simulink model "auto"  (R2024b)
settings: Solver=VariableStepAuto  StartTime=0.0  StopTime=10.0  RelTol=1e-3
undefined symbols (not defined in the file): control, controlParams, ControlSampleTime, Cruise_a, flightState, FSState, FWControlParams, FWTrimSpeed, uavParam, Vt, w_trim, zGround
libraries: slpidlib x21, simulink x6, uavalgslib x6
(part 1 of 4)
settings Model: Creator=USER  LastModifiedBy=USER

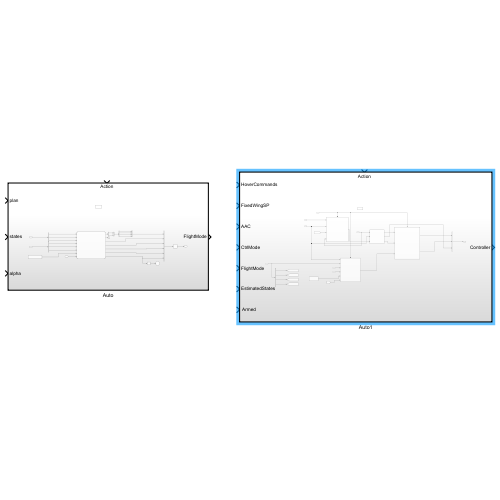
[thumbnail: Simulink's stored preview of the top-level diagram]
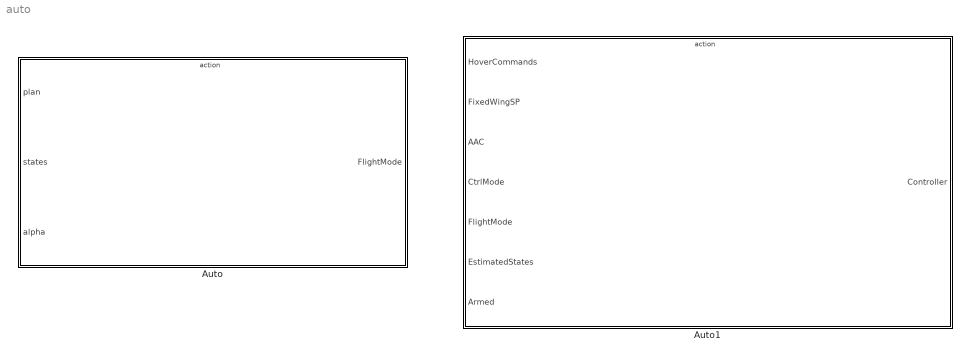
== system auto ==
  Auto : Subsystem  TreatAsAtomicUnit=on
  Auto1 : Subsystem  TreatAsAtomicUnit=on

== system auto/Auto ==
  plan : Inport  OutDataTypeStr=Bus: plan  SampleTime=0.005
  states : Inport  Port=2  OutDataTypeStr=Bus: states  SampleTime=0.005
  alpha : Inport  Port=3  SampleTime=0.005
  Action Port : ActionPort
  Bus Creator : BusCreator  Inputs=4  OutDataTypeStr=Bus: HoverSPBus
      settings: InheritFromInputs=off
  Bus Creator1 : BusCreator  Inputs=6  OutDataTypeStr=Bus: flightmode
  Bus Selector : BusSelector  OutputSignals=LAP,YawCmd
  Bus Selector1 : BusSelector  OutputSignals=mode,ToWP,FromWP
  Bus Selector2 : BusSelector  OutputSignals=pose,states,ground
  Compare To Constant : simulink/Logic and Bit Operations/Compare To Constant  relop===  const=2  OutDataTypeStr=boolean
  Constant2 : Constant  Value=FSState  SampleTime=-1
  Demux : Demux
  Guidance Mode Selector : Stateflow chart  TreatAsAtomicUnit=on
      settings: PortSchema="{\"entries\":[{\"content\":{\"sides\":[{\"content\":{\"connectorIds\":[\"In1\",\"In2\",\"In3\",\"In4\",\"In5\",\"In7\",\"In6\",\"In8\"]},\"type\":\"ConnectorPlacement.EquallySpacedRectSide\",\"uuid\":\"a9cfd0e2-196c-422d-b359-9161a47768c9\"},{\"content\":{\"connectorIds\":[\"Out7\",\"Out2\",\"Out4\",\"Out3\",\"Out5\",\"Out6\",\"Out1\"],\"side\":\"RIGHT\"},\"type\":\"ConnectorPlacement.EquallySpacedRectSide\",\"uuid\":\"4fed41ae-e7cf-4de3-8bdb-9e24e7d8b079\"},{\"content\":{\"side\":\"TOP\"},\"type\":\"ConnectorPlacement.EquallySpacedRectSide\",\"uuid\":\"2d49ff20-2f63-498d-ac9d-820eae01f794\"},{\"content\":{\"side\":\"BOTTOM\"},\"type\":\"ConnectorPlacement.EquallySpacedRectSide\",\"uuid\":\"da24ee44-6e15-4e50-9b36-ff21cb47946d\"}]},\"type\":\"ConnectorPlacement.EquallySpacedConnector\",\"uuid\":\"88d403f4-ad96-40f9-9697-84906f26a8bf\"}],\"packageUris\":[\"http://schema.mathworks.com/mf0/Connector/R2020b\"],\"version\":\"1.0\"}"
  Mux : Mux  Inputs=2
  Stop Simulation : Stop
  Terminator : Terminator
  Unit Delay : UnitDelay  SampleTime=-1  HasFrameUpgradeWarning=on
  FlightMode : Outport  OutDataTypeStr=Bus: flightmode
  wires:
  Bus Selector1/1 -> Guidance Mode Selector/1(mode)  "<mode>"
  Guidance Mode Selector/6(FlightMode) -> Bus Creator1/5  "FlightMode"
  Bus Selector1/3 -> Guidance Mode Selector/3(FromWP)  "<FromWP>"
  Bus Selector2/3 -> Guidance Mode Selector/7(Ground)  "<ground>"
  Bus Selector/1 -> Mux/1  "<LAP>"
  Guidance Mode Selector/5(controlMode) -> Bus Creator1/4  "controlMode"
  Guidance Mode Selector/3(aacSP) -> Bus Creator1/3  "AACSP"
  Guidance Mode Selector/7(InnerLoopCmds) -> Bus Selector/1
  Guidance Mode Selector/2(GdncMode) -> Terminator/1
  Bus Selector/2 -> Mux/2  "<YawCmd>"
  Compare To Constant/1 -> Stop Simulation/1
  Bus Selector2/2 -> Guidance Mode Selector/5(States)  "<states>"
  Mux/1 -> Demux/1
  Bus Selector2/1 -> Guidance Mode Selector/4(Pose)  "<pose>"
  Guidance Mode Selector/1(Status) -> Compare To Constant/1, Bus Creator1/6  "Status"
  Guidance Mode Selector/4(FixedWingSP) -> Bus Creator1/2  "FixedWingSP"
  Bus Selector1/2 -> Guidance Mode Selector/2(ToWP)  "<ToWP>"
  Demux/1 -> Bus Creator/1  "X"
  Demux/2 -> Bus Creator/2  "Y"
  Demux/3 -> Bus Creator/3  "Z"
  Demux/4 -> Bus Creator/4  "Yaw"
  Bus Creator/1 -> Bus Creator1/1  "HoverSP"
  Bus Creator1/1 -> Unit Delay/1
  alpha/1 -> Guidance Mode Selector/8(a)
  Constant2/1 -> Guidance Mode Selector/6(PresetMode)
  states/1 -> Bus Selector2/1
  plan/1 -> Bus Selector1/1
  Unit Delay/1 -> FlightMode/1

== system auto/Auto1 ==
  HoverCommands : Inport  OutDataTypeStr=Bus: HoverSPBus
  FixedWingSP : Inport  Port=2
  AAC : Inport  Port=3
  CtrlMode : Inport  Port=4
  FlightMode : Inport  Port=5
  EstimatedStates : Inport  Port=6
  " Armed" : Inport  Port=7
  Action Port : ActionPort
  Blend Scheduler : Subsystem
  Bus Creator : BusCreator  Inputs=3  OutDataTypeStr=Bus: controller
  Bus Selector2 : BusSelector  OutputSignals=inTransition,TransitionCondition,BackTransitionCondition,TransitionStep
  Fixed Wing Controller : Subsystem  TreatAsAtomicUnit=on  VariantControl=Fixed Wing Controller
  Manual Control : Subsystem
  Multicopter Controller : Subsystem  TreatAsAtomicUnit=on
  Scheduler : Subsystem  SystemSampleTime=0.005
  Controller : Outport
  wires:
  Scheduler/1(MotorActuatorCommands) -> Bus Creator/1  "MotorActuatorCommands"
  Manual Control/1(AERT) -> Fixed Wing Controller/5(AERT)
  Scheduler/2(CtrlSurfaceCommands) -> Bus Creator/2  "CtrlSurfaceCommands"
  Fixed Wing Controller/1(Actuator) -> Scheduler/3(FixedWingActuators)
  Blend Scheduler/2(alpha) -> Bus Creator/3  "a"
  Multicopter Controller/1(MixerCommands) -> Blend Scheduler/3(MixerCommands)
  AAC/1 -> Fixed Wing Controller/3(AAC SP)
  FixedWingSP/1 -> Fixed Wing Controller/4(FixedWingSP)
  [InTransition] -> Multicopter Controller/3(InTransition)
  " Armed"/1 -> Fixed Wing Controller/Enable, Scheduler/Enable, Multicopter Controller/Enable
  HoverCommands/1 -> Multicopter Controller/1(Hover Commands)
  EstimatedStates/1 -> Fixed Wing Controller/1(States), Blend Scheduler/2(States), Multicopter Controller/2(States)
  FlightMode/1 -> Multicopter Controller/4(FlightMode), Blend Scheduler/1(FlightMode)
  Bus Selector2/2 -> [TransitionDone]  "<TransitionCondition>"
  CtrlMode/1 -> Bus Selector2/1, Fixed Wing Controller/2(Control Mode)
  Bus Selector2/1 -> [InTransition]  "<inTransition>"
  Bus Selector2/3 -> [BackTransitionDone]  "<BackTransitionCondition>"
  Bus Creator/1 -> Controller/1
  Blend Scheduler/3(FlightState) -> Scheduler/2(FlightState)
  [InTransition] -> Fixed Wing Controller/6(In1)
  Bus Selector2/4 -> [TransitionStep]  "<TransitionStep>"
  Blend Scheduler/1(MotorCommands) -> Scheduler/1(MotorCommands)

== system auto/Auto/Guidance Mode Selector/GuidanceLogic.BackTransition ==
  States : Inport  OutDataTypeStr=Bus: GuidanceStates
  Action Port : ActionPort
      settings: CopyFcn=Stateflow.SLINSF.SimulinkMan.removeBlockPreDeleteFcn  PreDeleteFcn=Stateflow.SLINSF.SimulinkMan.unsafePredeleteFcn
  Bus Creator1 : BusCreator  Inputs=3  OutDataTypeStr=Bus: innerLoopCmdsBus  NonVirtualBus=on
  Bus Selector : BusSelector  OutputSignals=Xe
  Constant : Constant  Value=0
  Constant1 : Constant  Value=0
  Constant2 : Constant  Value=0
  Data Type Conversion : DataTypeConversion  OutDataTypeStr=uint8  SaturateOnIntegerOverflow=off  RndMeth=Floor
  Gain : Gain
  Status : Outport
  InnerLoopCmds : Outport  Port=2  OutDataTypeStr=Bus: innerLoopCmdsBus
  wires:
  States/1 -> Bus Selector/1
  Bus Selector/1 -> Gain/1  "<Xe>"
  Bus Creator1/1 -> InnerLoopCmds/1
  Constant1/1 -> Bus Creator1/2  "HeadingCmd"
  Constant2/1 -> Bus Creator1/3  "YawCmd"
  Data Type Conversion/1 -> Status/1
  Gain/1 -> Bus Creator1/1  "LAP"
  Constant/1 -> Data Type Conversion/1

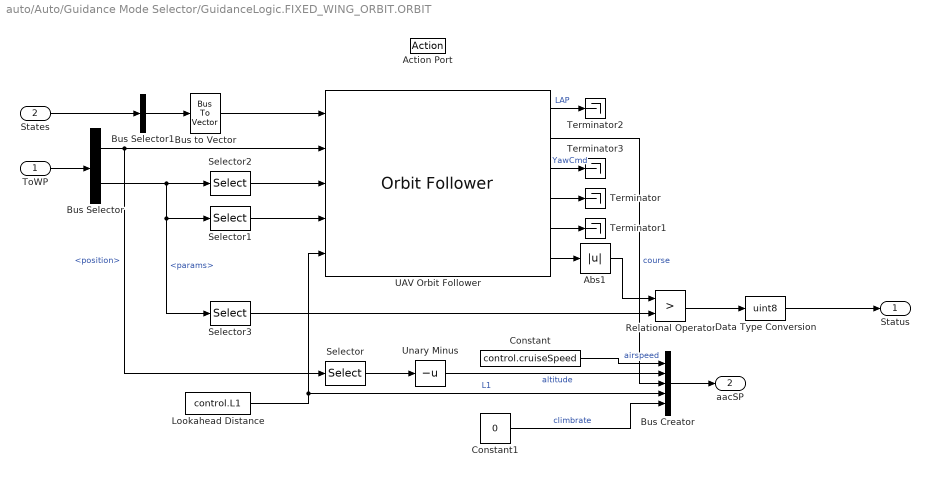
== system auto/Auto/Guidance Mode Selector/GuidanceLogic.FIXED_WING_ORBIT.ORBIT ==
  ToWP : Inport  OutDataTypeStr=Bus: UAVPathManagerBus
  States : Inport  Port=2
  Action Port : ActionPort
      settings: CopyFcn=Stateflow.SLINSF.SimulinkMan.removeBlockPreDeleteFcn  PreDeleteFcn=Stateflow.SLINSF.SimulinkMan.unsafePredeleteFcn
  Abs1 : Abs  SaturateOnIntegerOverflow=off
  Bus Creator : BusCreator  Inputs=5  OutDataTypeStr=Bus: AAC  NonVirtualBus=on
      settings: InheritFromInputs=off
  Bus Selector : BusSelector  OutputSignals=position,params
  Bus Selector1 : BusSelector  OutputSignals=Xe,course  OutputAsBus=on
  Bus to Vector : BusToVector
  Constant : Constant  Value=control.cruiseSpeed
  Constant1 : Constant  Value=0
  Data Type Conversion : DataTypeConversion  OutDataTypeStr=uint8  SaturateOnIntegerOverflow=off  RndMeth=Floor
  Lookahead Distance : Constant  Value=control.L1  OutDataTypeStr=double
  Relational Operator : RelationalOperator  Operator=>  OutDataTypeStr=boolean  RndMeth=Simplest  InputSameDT=off
  Selector : Selector  InputPortWidth=3  IndexOptions=Index vector (dialog)  Indices=3  OutputSizes=1
  Selector1 : Selector  InputPortWidth=4  IndexOptions=Index vector (dialog)  Indices=2  OutputSizes=1
  Selector2 : Selector  InputPortWidth=4  IndexOptions=Index vector (dialog)  Indices=1  OutputSizes=1
  Selector3 : Selector  InputPortWidth=4  IndexOptions=Index vector (dialog)  Indices=3  OutputSizes=1
  Terminator{,1..3} (4 alike) : Terminator
  UAV Orbit Follower : uavalgslib/Orbit Follower  UAVType=fixed-wing  MinOrbitRadius=control.turningRadius  MinLookaheadDistance=control.L1  ExternalReset=none  ShowCrossTrackErrorOutput=off  ShowNumTurnsOutput=on  SimulateUsing=Code generation
  Unary Minus : UnaryMinus
  Status : Outport
  aacSP : Outport  Port=2
  wires:
  Bus to Vector/1 -> UAV Orbit Follower/1
  Selector2/1 -> UAV Orbit Follower/3
  Bus Selector/1 -> UAV Orbit Follower/2, Selector/1  "<position>"
  ToWP/1 -> Bus Selector/1
  Bus Selector/2 -> Selector1/1, Selector3/1, Selector2/1  "<params>"
  Selector3/1 -> Relational Operator/2
  Relational Operator/1 -> Data Type Conversion/1
  UAV Orbit Follower/4 -> Terminator/1
  UAV Orbit Follower/5 -> Terminator1/1
  Bus Selector1/1 -> Bus to Vector/1
  States/1 -> Bus Selector1/1
  UAV Orbit Follower/1 -> Terminator2/1  "LAP"
  Lookahead Distance/1 -> UAV Orbit Follower/5, Bus Creator/4  "L1"
  Bus Creator/1 -> aacSP/1
  UAV Orbit Follower/2 -> Bus Creator/3  "course"
  Constant/1 -> Bus Creator/1  "airspeed"
  Unary Minus/1 -> Bus Creator/2  "altitude"
  UAV Orbit Follower/3 -> Terminator3/1  "YawCmd"
  Selector/1 -> Unary Minus/1
  UAV Orbit Follower/6 -> Abs1/1
  Abs1/1 -> Relational Operator/1
  Selector1/1 -> UAV Orbit Follower/4
  Constant1/1 -> Bus Creator/5  "climbrate"
  Data Type Conversion/1 -> Status/1

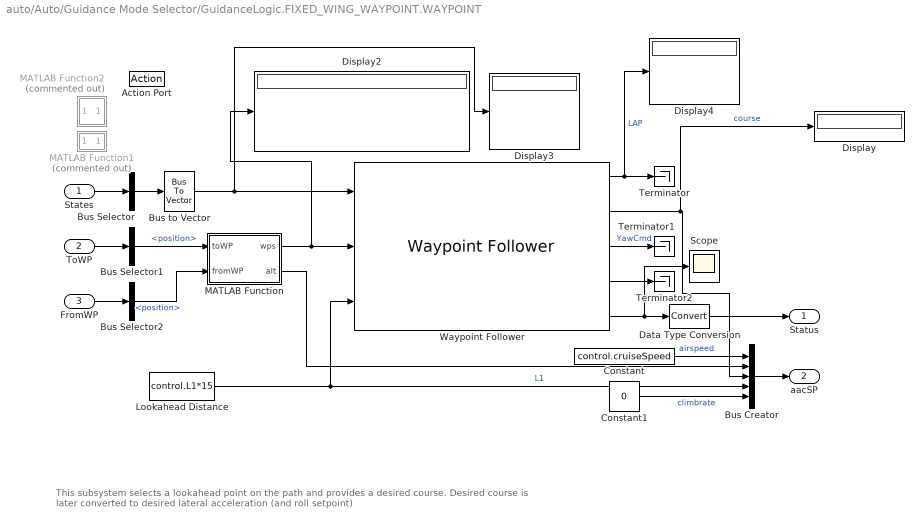
== system auto/Auto/Guidance Mode Selector/GuidanceLogic.FIXED_WING_WAYPOINT.WAYPOINT ==
  note: This subsystem selects a lookahead point on the path and provides a desired course. Desired course is later converted to desired lateral acceleration (and roll setpoint)
  States : Inport  OutDataTypeStr=Bus: GuidanceStates
  ToWP : Inport  Port=2  OutDataTypeStr=Bus: UAVPathManagerBus
  FromWP : Inport  Port=3  OutDataTypeStr=Bus: UAVPathManagerBus
  Action Port : ActionPort
      settings: CopyFcn=Stateflow.SLINSF.SimulinkMan.removeBlockPreDeleteFcn  PreDeleteFcn=Stateflow.SLINSF.SimulinkMan.unsafePredeleteFcn
  Bus Creator : BusCreator  Inputs=5  OutDataTypeStr=Bus: AAC  NonVirtualBus=on
      settings: InheritFromInputs=off
  Bus Selector : BusSelector  OutputSignals=Xe,course  OutputAsBus=on
  Bus Selector1 : BusSelector  OutputSignals=position
  Bus Selector2 : BusSelector  OutputSignals=position
  Bus to Vector : BusToVector
  Constant : Constant  Value=control.cruiseSpeed
  Constant1 : Constant  Value=0
  Data Type Conversion : DataTypeConversion  SaturateOnIntegerOverflow=off  RndMeth=Floor
  Display{,2..4} (4 alike) : Display
  Lookahead Distance : Constant  Value=control.L1*15  OutDataTypeStr=double
  MATLAB Function : MATLAB Function  TreatAsAtomicUnit=on
  MATLAB Function1 : MATLAB Function  Commented=on  TreatAsAtomicUnit=on
  MATLAB Function2 : MATLAB Function  Commented=on  TreatAsAtomicUnit=on
  Scope : Scope
  Terminator : Terminator
  Terminator1 : Terminator
  Terminator2 : Terminator
  Waypoint Follower : uavalgslib/Waypoint Follower  UAVType=fixed-wing  StartFrom=first  TransitionRadiusSource=internal  TransitionRadius=FWControl.transitionRadius  MinLookaheadDistance=control.L1  HoverAtLastWaypoint=off  YawInput=off  ShowCrossTrackErrorOutput=off  ShowStatusOutput=on  SimulateUsing=Code generation
  Status : Outport
  aacSP : Outport  Port=2
  wires:
  Lookahead Distance/1 -> Waypoint Follower/3, Bus Creator/4  "L1"
  Waypoint Follower/1 -> Display4/1, Terminator/1  "LAP"
  Waypoint Follower/3 -> Terminator1/1  "YawCmd"
  Waypoint Follower/4 -> Terminator2/1
  Constant/1 -> Bus Creator/1  "airspeed"
  States/1 -> Bus Selector/1
  Bus Selector/1 -> Bus to Vector/1
  Waypoint Follower/5 -> Scope/1, Data Type Conversion/1
  Data Type Conversion/1 -> Status/1
  Bus Creator/1 -> aacSP/1
  ToWP/1 -> Bus Selector1/1
  FromWP/1 -> Bus Selector2/1
  Bus Selector1/1 -> MATLAB Function/1(toWP)  "<position>"
  Bus Selector2/1 -> MATLAB Function/2(fromWP)  "<position>"
  MATLAB Function/2(alt) -> Bus Creator/2
  Waypoint Follower/2 -> Display/1, Bus Creator/3  "course"
  Constant1/1 -> Bus Creator/5  "climbrate"
  Bus to Vector/1 -> Display3/1, Waypoint Follower/1
  MATLAB Function/1(wps) -> Display2/1, Waypoint Follower/2

== system auto/Auto/Guidance Mode Selector/GuidanceLogic.ForwardTransition ==
  ToWP : Inport  OutDataTypeStr=Bus: UAVPathManagerBus
  FromWP : Inport  Port=2  OutDataTypeStr=Bus: UAVPathManagerBus
  Action Port : ActionPort
      settings: CopyFcn=Stateflow.SLINSF.SimulinkMan.removeBlockPreDeleteFcn  PreDeleteFcn=Stateflow.SLINSF.SimulinkMan.unsafePredeleteFcn
  Bus Creator : BusCreator  Inputs=5  OutDataTypeStr=Bus: AAC  NonVirtualBus=on
      settings: InheritFromInputs=off
  Bus Creator1 : BusCreator  Inputs=3  OutDataTypeStr=Bus: innerLoopCmdsBus  NonVirtualBus=on
  Bus Selector1 : BusSelector  OutputSignals=position
  Bus Selector2 : BusSelector  OutputSignals=position
  Constant : Constant  Value=0
  Constant1 : Constant  Value=0
  Constant2 : Constant  Value=0
  Constant3 : Constant  Value=[0 0 0]
  Data Type Conversion : DataTypeConversion  OutDataTypeStr=uint8  SaturateOnIntegerOverflow=off  RndMeth=Floor
  MATLAB Function : MATLAB Function  TreatAsAtomicUnit=on
  Switch : Switch  Criteria=u2 > Threshold  SaturateOnIntegerOverflow=off  InputSameDT=off
  Terminator : Terminator
  Status : Outport
  InnerLoopCmds : Outport  Port=2  OutDataTypeStr=Bus: innerLoopCmdsBus
  aacSP : Outport  Port=3
  wires:
  Bus Creator1/1 -> InnerLoopCmds/1
  Constant1/1 -> Bus Creator1/2  "HeadingCmd"
  Constant2/1 -> Bus Creator1/3  "YawCmd"
  Data Type Conversion/1 -> Status/1
  Constant/1 -> Data Type Conversion/1
  Constant3/1 -> Bus Creator1/1  "LAP"
  FromWP/1 -> Bus Selector2/1
  Bus Selector1/1 -> MATLAB Function/1(toWP)  "<position>"
  Bus Selector2/1 -> MATLAB Function/2(fromWP)  "<position>"
  ToWP/1 -> Bus Selector1/1
  Bus Creator/1 -> aacSP/1
  MATLAB Function/1(wps) -> Terminator/1
  MATLAB Function/2(alt) -> Bus Creator/2  "alt"

== system auto/Auto/Guidance Mode Selector/GuidanceLogic.Land.Descend ==
  ToWP : Inport  OutDataTypeStr=Bus: UAVPathManagerBus
  Ground : Inport  Port=2
  Pose : Inport  Port=3
  FromWP : Inport  Port=4  OutDataTypeStr=Bus: UAVPathManagerBus
  Action Port : ActionPort
      settings: CopyFcn=Stateflow.SLINSF.SimulinkMan.removeBlockPreDeleteFcn  PreDeleteFcn=Stateflow.SLINSF.SimulinkMan.unsafePredeleteFcn
  Bus Creator : BusCreator  Inputs=3  OutDataTypeStr=Bus: innerLoopCmdsBus  NonVirtualBus=on
      settings: InheritFromInputs=off
  Bus Selector : BusSelector  OutputSignals=position,params
  Constant : Constant  Value=3
  Constant3 : Constant  Value=0  OutDataTypeStr=uint8
  Hdg Cmd Sat : Saturate  UpperLimit=pi  LowerLimit=-pi
      settings: AttributesFormatString=[%<UpperLimit> %<LowerLimit>]
  MATLAB Function : MATLAB Function  TreatAsAtomicUnit=on
  Mux : Mux  Inputs=2
  Selector : Selector  InputPortWidth=3  IndexOptions=Index vector (dialog)  Indices=[1 2]  OutputSizes=1
  Selector1 : Selector  InputPortWidth=4  IndexOptions=Index vector (dialog)  Indices=4  OutputSizes=1
  Selector3 : Selector  InputPortWidth=4  IndexOptions=Index vector (dialog)  Indices=4  OutputSizes=1
  Waypoint Follower : uavalgslib/Waypoint Follower  UAVType=multirotor  StartFrom=first  TransitionRadiusSource=internal  TransitionRadius=1  MinLookaheadDistance=0.1  HoverAtLastWaypoint=on  YawInput=on  ShowCrossTrackErrorOutput=off  ShowStatusOutput=off  SimulateUsing=Code generation
  Yaw Cmd Sat : Saturate  UpperLimit=pi  LowerLimit=-pi
      settings: AttributesFormatString=[%<UpperLimit> %<LowerLimit>]
  InnerLoopCmds : Outport  OutDataTypeStr=Bus: innerLoopCmdsBus
  Status : Outport  Port=2
  wires:
  Bus Creator/1 -> InnerLoopCmds/1
  Bus Selector/1 -> Selector/1  "<position>"
  Yaw Cmd Sat/1 -> Bus Creator/3  "YawCmd"
  Hdg Cmd Sat/1 -> Bus Creator/2  "HeadingCmd"
  ToWP/1 -> Bus Selector/1
  Selector1/1 -> Yaw Cmd Sat/1
  Selector3/1 -> Hdg Cmd Sat/1
  Selector/1 -> Mux/1  "LAP"
  Bus Selector/2 -> MATLAB Function/3(ToWPParam), Selector1/1, Selector3/1  "<params>"
  Ground/1 -> Mux/2
  Constant3/1 -> Status/1
  Mux/1 -> MATLAB Function/2(ToWPPos)  "LAP"
  FromWP/1 -> MATLAB Function/1(FromWP)
  Pose/1 -> Waypoint Follower/1
  MATLAB Function/1(wps) -> Waypoint Follower/2
  Constant/1 -> Waypoint Follower/3
  Waypoint Follower/1 -> Bus Creator/1  "LAP"

== system auto/Auto/Guidance Mode Selector/GuidanceLogic.Land.ToLand ==
  Pose : Inport
  ToWP : Inport  Port=2  OutDataTypeStr=Bus: UAVPathManagerBus
  FromWP : Inport  Port=3  OutDataTypeStr=Bus: UAVPathManagerBus
  Action Port : ActionPort
      settings: CopyFcn=Stateflow.SLINSF.SimulinkMan.removeBlockPreDeleteFcn  PreDeleteFcn=Stateflow.SLINSF.SimulinkMan.unsafePredeleteFcn
  Bus Creator1 : BusCreator  Inputs=3  OutDataTypeStr=Bus: innerLoopCmdsBus  NonVirtualBus=on
  Constant : Constant  Value=0  OutDataTypeStr=uint8
  Lookahead Distance : Constant  Value=10  OutDataTypeStr=double
  MATLAB Function : MATLAB Function  TreatAsAtomicUnit=on
  Scope : Scope
  Waypoint Follower : uavalgslib/Waypoint Follower  UAVType=multirotor  StartFrom=first  TransitionRadiusSource=internal  TransitionRadius=1  MinLookaheadDistance=0.1  HoverAtLastWaypoint=on  YawInput=on  ShowCrossTrackErrorOutput=off  ShowStatusOutput=off  SimulateUsing=Code generation
  Status : Outport
  InnerLoopCmds : Outport  Port=2  OutDataTypeStr=Bus: innerLoopCmdsBus
  wires:
  Constant/1 -> Status/1
  MATLAB Function/1(wps) -> Waypoint Follower/2
  Lookahead Distance/1 -> Waypoint Follower/3
  Bus Creator1/1 -> InnerLoopCmds/1
  ToWP/1 -> MATLAB Function/2(ToWP)
  Waypoint Follower/2 -> Bus Creator1/2  "HeadingCmd"
  FromWP/1 -> MATLAB Function/1(FromWP)
  Waypoint Follower/4 -> Scope/1
  Pose/1 -> Waypoint Follower/1
  Waypoint Follower/3 -> Bus Creator1/3  "YawCmd"
  Waypoint Follower/1 -> Bus Creator1/1  "LAP"

== system auto/Auto/Guidance Mode Selector/GuidanceLogic.Orbit ==
  ToWP : Inport  OutDataTypeStr=Bus: UAVPathManagerBus
  Pose : Inport  Port=2
  Action Port : ActionPort
      settings: CopyFcn=Stateflow.SLINSF.SimulinkMan.removeBlockPreDeleteFcn  PreDeleteFcn=Stateflow.SLINSF.SimulinkMan.unsafePredeleteFcn
  Abs : Abs  SaturateOnIntegerOverflow=off
  Bus Creator : BusCreator  Inputs=3  OutDataTypeStr=Bus: innerLoopCmdsBus  NonVirtualBus=on
  Bus Selector : BusSelector  OutputSignals=position,params
  Data Type Conversion : DataTypeConversion  OutDataTypeStr=uint8  SaturateOnIntegerOverflow=off  RndMeth=Floor
  Lookahead Distance : Constant  Value=5  OutDataTypeStr=double
  Radius : Selector  InputPortWidth=4  IndexOptions=Index vector (dialog)  Indices=[3]  OutputSizes=1
  Relational Operator : RelationalOperator  Operator=>  OutDataTypeStr=boolean  RndMeth=Simplest  InputSameDT=off
  Sign : Signum  ZeroCross=off
  Terminator : Terminator
  Terminator1 : Terminator
  Turns : Selector  InputPortWidth=4  IndexOptions=Index vector (dialog)  Indices=[1]  OutputSizes=1
  UAV Orbit Follower : uavalgslib/Orbit Follower  UAVType=multirotor  MinOrbitRadius=1  MinLookaheadDistance=0.1  ExternalReset=none  ShowCrossTrackErrorOutput=off  ShowNumTurnsOutput=on  SimulateUsing=Code generation
  InnerLoopCmds : Outport  OutDataTypeStr=Bus: innerLoopCmdsBus
  Status : Outport  Port=2
  wires:
  Pose/1 -> UAV Orbit Follower/1
  Lookahead Distance/1 -> UAV Orbit Follower/5
  Abs/1 -> UAV Orbit Follower/3
  Bus Selector/1 -> UAV Orbit Follower/2  "<position>"
  ToWP/1 -> Bus Selector/1
  Bus Creator/1 -> InnerLoopCmds/1
  UAV Orbit Follower/2 -> Bus Creator/2  "HeadingCmd"
  UAV Orbit Follower/3 -> Bus Creator/3  "YawCmd"
  Bus Selector/2 -> Turns/1, Radius/1  "<params>"
  Radius/1 -> Abs/1, Sign/1
  Sign/1 -> UAV Orbit Follower/4
  Relational Operator/1 -> Data Type Conversion/1
  Turns/1 -> Relational Operator/2
  Data Type Conversion/1 -> Status/1
  UAV Orbit Follower/6 -> Relational Operator/1
  UAV Orbit Follower/4 -> Terminator/1
  UAV Orbit Follower/5 -> Terminator1/1
  UAV Orbit Follower/1 -> Bus Creator/1  "LAP"

== system auto/Auto/Guidance Mode Selector/GuidanceLogic.Takeoff ==
  ToWP : Inport  OutDataTypeStr=Bus: UAVPathManagerBus
  Pose : Inport  Port=2
  Action Port : ActionPort
      settings: CopyFcn=Stateflow.SLINSF.SimulinkMan.removeBlockPreDeleteFcn  PreDeleteFcn=Stateflow.SLINSF.SimulinkMan.unsafePredeleteFcn
  Bus Creator : BusCreator  Inputs=3  OutDataTypeStr=Bus: innerLoopCmdsBus  NonVirtualBus=on
      settings: InheritFromInputs=off
  Bus Selector : BusSelector  OutputSignals=position,params
  Constant : Constant  Value=0  OutDataTypeStr=uint8
  Constant1 : Constant  Value=0
  Demux : Demux  Outputs=[2 2]
  Demux1 : Demux  Outputs=[2 1]
  Hdg. Cmd Sat : Saturate  UpperLimit=pi  LowerLimit=-pi
      settings: AttributesFormatString=[%<UpperLimit> %<LowerLimit>]
  Mux : Mux  Inputs=2
  Selector3 : Selector  InputPortWidth=4  IndexOptions=Index vector (dialog)  Indices=4  OutputSizes=1
  Terminator : Terminator
  Terminator1 : Terminator
  Yaw Cmd Sat : Saturate  UpperLimit=pi  LowerLimit=-pi
      settings: AttributesFormatString=[%<UpperLimit> %<LowerLimit>]
  InnerLoopCmds : Outport  OutDataTypeStr=Bus: innerLoopCmdsBus
  Status : Outport  Port=2
  wires:
  Hdg. Cmd Sat/1 -> Bus Creator/2  "HeadingCmd"
  Bus Creator/1 -> InnerLoopCmds/1
  Constant/1 -> Status/1
  Pose/1 -> Demux/1
  Yaw Cmd Sat/1 -> Bus Creator/3  "YawCmd"
  ToWP/1 -> Bus Selector/1
  Bus Selector/2 -> Selector3/1  "<params>"
  Demux/1 -> Mux/1
  Bus Selector/1 -> Demux1/1  "<position>"
  Demux/2 -> Terminator/1
  Demux1/1 -> Terminator1/1
  Selector3/1 -> Hdg. Cmd Sat/1
  Constant1/1 -> Yaw Cmd Sat/1
  Demux1/2 -> Mux/2
  Mux/1 -> Bus Creator/1  "LAP"

== system auto/Auto/Guidance Mode Selector/GuidanceLogic.WP ==
  FromWP : Inport  OutDataTypeStr=Bus: UAVPathManagerBus
  Pose : Inport  Port=2
  ToWP : Inport  Port=3  OutDataTypeStr=Bus: UAVPathManagerBus
  Action Port : ActionPort
      settings: CopyFcn=Stateflow.SLINSF.SimulinkMan.removeBlockPreDeleteFcn  PreDeleteFcn=Stateflow.SLINSF.SimulinkMan.unsafePredeleteFcn
  Back Transition Guard : Subsystem
  Bus Creator : BusCreator  Inputs=3  OutDataTypeStr=Bus: innerLoopCmdsBus  NonVirtualBus=on
  Bus Creator1 : BusCreator  Inputs=1
  Bus Creator2 : BusCreator  Inputs=3
  Bus Selector : BusSelector  OutputSignals=position
  Constant1 : Constant
  Data Type Conversion : DataTypeConversion  OutDataTypeStr=uint8  SaturateOnIntegerOverflow=off  RndMeth=Floor
  Data Type Conversion1 : DataTypeConversion  OutDataTypeStr=double  SaturateOnIntegerOverflow=off  RndMeth=Floor
  Data Type Conversion2 : DataTypeConversion  OutDataTypeStr=double  SaturateOnIntegerOverflow=off  RndMeth=Floor
  Demux : Demux  Outputs=3
  Dist2WP : Subsystem
  Lookahead Distance : Constant  Value=10  OutDataTypeStr=double
  MATLAB Function : MATLAB Function  TreatAsAtomicUnit=on
  Relational Operator : RelationalOperator  OutDataTypeStr=boolean  RndMeth=Simplest  InputSameDT=off
  Scope : Scope
  Selector : Selector  InputPortWidth=3  IndexOptions=Index vector (dialog)  Indices=3  OutputSizes=1
  Terminator1 : Terminator
  Waypoint Follower : uavalgslib/Waypoint Follower  UAVType=multirotor  StartFrom=closest  TransitionRadiusSource=internal  TransitionRadius=R_WAYPOINTTRANSITION  MinLookaheadDistance=0.1  HoverAtLastWaypoint=off  YawInput=on  ShowCrossTrackErrorOutput=off  ShowStatusOutput=off  SimulateUsing=Code generation
  Yaw Cmd Sat : Saturate  UpperLimit=pi  LowerLimit=-pi
      settings: AttributesFormatString=[%<UpperLimit> %<LowerLimit>]
  InnerLoopCmds : Outport  OutDataTypeStr=Bus: innerLoopCmdsBus
  Status : Outport  Port=2
  wires:
  Data Type Conversion/1 -> Status/1
  Bus Creator/1 -> InnerLoopCmds/1
  ToWP/1 -> Dist2WP/3(ToWP), Bus Selector/1, MATLAB Function/2(ToWP)
  MATLAB Function/1(wps) -> Waypoint Follower/2
  Waypoint Follower/2 -> Bus Creator/2  "HeadingCmd"
  Waypoint Follower/4 -> Scope/1
  Dist2WP/1(Dist) -> Relational Operator/2
  FromWP/1 -> Back Transition Guard/2(FromWP)
  Relational Operator/1 -> Data Type Conversion/1
  Back Transition Guard/1(PrevWP) -> Dist2WP/2(FromWP), MATLAB Function/1(FromWP)
  Pose/1 -> Back Transition Guard/1(Poses), Waypoint Follower/1, Dist2WP/1(Pose)
  Lookahead Distance/1 -> Waypoint Follower/3
  Waypoint Follower/3 -> Yaw Cmd Sat/1  "YawCmd"
  Yaw Cmd Sat/1 -> Bus Creator/3  "YawCmd"
  Constant1/1 -> Relational Operator/1
  Bus Creator1/1 -> Data Type Conversion1/1  "LAP"
  Waypoint Follower/1 -> Demux/1  "LAP"
  Demux/3 -> Terminator1/1
  Data Type Conversion1/1 -> Selector/1  "LAP"
  Selector/1 -> Bus Creator2/3  "Z"
  Demux/1 -> Bus Creator2/1  "X"
  Demux/2 -> Bus Creator2/2  "Y"
  Bus Creator2/1 -> Data Type Conversion2/1  "LAP"
  Data Type Conversion2/1 -> Bus Creator/1  "LAP"
  Bus Selector/1 -> Bus Creator1/1  "<position>"

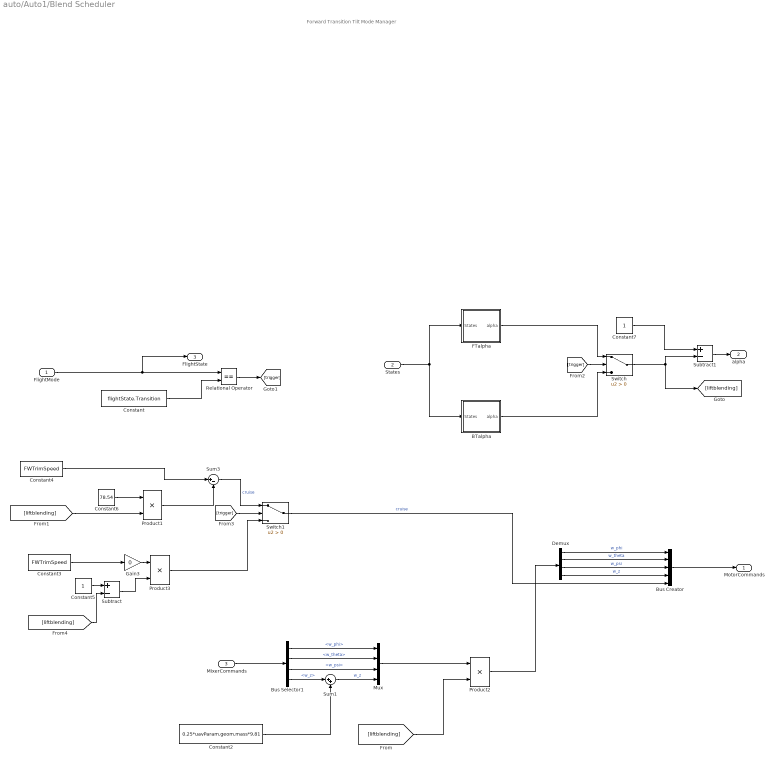
== system auto/Auto1/Blend Scheduler ==
  note: Forward Transition Tilt Mode Manager
  FlightMode : Inport
  States : Inport  Port=2
  MixerCommands : Inport  Port=3
  BTalpha : Subsystem  TreatAsAtomicUnit=on
  Bus Creator : BusCreator  Inputs=5
  Bus Selector1 : BusSelector  OutputSignals=w_phi,w_theta,w_psi,w_z
  Constant : Constant  Value=flightState.Transition
  Constant2 : Constant  Value=0.25*uavParam.geom.mass*9.81
  Constant3 : Constant  Value=FWTrimSpeed
  Constant4 : Constant  Value=FWTrimSpeed
  Constant5 : Constant
  Constant6 : Constant  Value=78.54
  Constant7 : Constant
  Demux : Demux
  FTalpha : Subsystem
  Gain3 : Gain  Gain=0
  Mux : Mux
  Product1 : Product
  Product2 : Product
  Product3 : Product
  Relational Operator : RelationalOperator  Operator===  OutDataTypeStr=boolean  RndMeth=Simplest  InputSameDT=off
  Subtract : Sum  Inputs=+-
  Subtract1 : Sum  Inputs=+-
  Sum1 : Sum  Inputs=|++
  Sum3 : Sum  Inputs=|+-
  Switch : Switch  Criteria=u2 > Threshold  SaturateOnIntegerOverflow=off  InputSameDT=off
  Switch1 : Switch  Criteria=u2 > Threshold  SaturateOnIntegerOverflow=off  InputSameDT=off
  MotorCommands : Outport
  alpha : Outport  Port=2
  FlightState : Outport  Port=3
  wires:
  FlightMode/1 -> Relational Operator/1, FlightState/1
  Relational Operator/1 -> [trigger]
  Bus Selector1/4 -> Sum1/1  "<w_z>"
  Constant2/1 -> Sum1/2
  [liftblending] -> Product2/2
  Mux/1 -> Product2/1
  MixerCommands/1 -> Bus Selector1/1
  Bus Selector1/1 -> Mux/1  "<w_phi>"
  Bus Selector1/2 -> Mux/2  "<w_theta>"
  Bus Selector1/3 -> Mux/3  "<w_psi>"
  Sum1/1 -> Mux/4  "w_z"
  Product2/1 -> Demux/1
  Demux/1 -> Bus Creator/1  "w_phi"
  Demux/2 -> Bus Creator/2  "w_theta"
  Demux/3 -> Bus Creator/3  "w_psi"
  Demux/4 -> Bus Creator/4  "w_z"
  Bus Creator/1 -> MotorCommands/1
  Constant6/1 -> Product1/1
  States/1 -> FTalpha/1(States), BTalpha/1(States)
  Switch/1 -> [liftblending], Subtract1/2
  FTalpha/1(alpha) -> Switch/1
  BTalpha/1(alpha) -> Switch/3
  [trigger] -> Switch/2
  Product1/1 -> Sum3/2
  Sum3/1 -> Switch1/1  "cruise"
  [trigger] -> Switch1/2
  Switch1/1 -> Bus Creator/5  "cruise"
  Constant3/1 -> Gain3/1
  Gain3/1 -> Product3/1
  Constant5/1 -> Subtract/1
  [liftblending] -> Subtract/2
  Subtract/1 -> Product3/2
  Product3/1 -> Switch1/3
  Constant7/1 -> Subtract1/1
  Subtract1/1 -> alpha/1
  Constant/1 -> Relational Operator/2
  [liftblending] -> Product1/2
  Constant4/1 -> Sum3/1

== system auto/Auto1/Fixed Wing Controller ==
  States : Inport
  Control Mode : Inport  Port=2
  AAC SP : Inport  Port=3  OutDataTypeStr=Bus: AAC
  FixedWingSP : Inport  Port=4  OutDataTypeStr=Bus: FixedWingCommandBus
  AERT : Inport  Port=5
  In1 : Inport  Port=6
  Actuator Armed : EnablePort
  Subsystem : Subsystem
  Actuator : Outport
  wires:
  States/1 -> Subsystem/1(States)
  Control Mode/1 -> Subsystem/2(Control Mode)
  AAC SP/1 -> Subsystem/3(AAC SP)
  Subsystem/1(Actuator) -> Actuator/1
  AERT/1 -> Subsystem/5(AERT)
  FixedWingSP/1 -> Subsystem/4(FixedWingSP)
  In1/1 -> Subsystem/6(Intransition)

== system auto/Auto1/Manual Control ==
  Bus Creator : BusCreator  Inputs=4
  Constant{,1..3} (4 alike) : Constant  Value=0  SampleTime=-1
  AERT : Outport
  wires:
  Constant/1 -> Bus Creator/1  "aileron"
  Constant1/1 -> Bus Creator/2  "throttle"
  Constant2/1 -> Bus Creator/3  "elevator"
  Constant3/1 -> Bus Creator/4  "rudder"
  Bus Creator/1 -> AERT/1

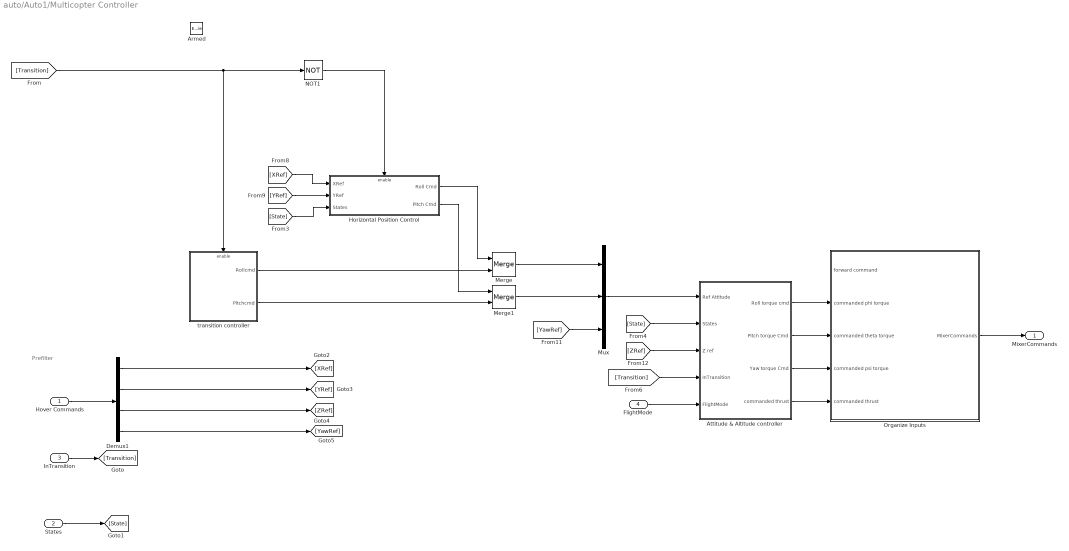
== system auto/Auto1/Multicopter Controller ==
  note: Prefilter
  Hover Commands : Inport  OutDataTypeStr=Bus: HoverSPBus
  States : Inport  Port=2
  InTransition : Inport  Port=3
  FlightMode : Inport  Port=4
  " Armed" : EnablePort
  Attitude & Altitude controller : Subsystem
  Demux1 : Demux
  Horizontal Position Control : Subsystem  TreatAsAtomicUnit=on
  Merge : Merge
  Merge1 : Merge
  Mux : Mux  Inputs=3
  NOT1 : Logic  Operator=NOT  IconShape=distinctive  AllPortsSameDT=off  OutDataTypeStr=boolean
  Organize Inputs : Subsystem
  transition controller : Subsystem
  MixerCommands : Outport
  wires:
  Organize Inputs/1(MixerCommands) -> MixerCommands/1
  Demux1/1 -> [XRef]
  [State] -> Horizontal Position Control/3(States)
  Demux1/3 -> [ZRef]
  NOT1/1 -> Horizontal Position Control/Enable
  [XRef] -> Horizontal Position Control/1(XRef)
  [YRef] -> Horizontal Position Control/2(YRef)
  InTransition/1 -> [Transition]
  States/1 -> [State]
  Hover Commands/1 -> Demux1/1
  Demux1/4 -> [YawRef]
  Mux/1 -> Attitude & Altitude controller/1(Ref Attitude)
  [State] -> Attitude & Altitude controller/2(States)
  [ZRef] -> Attitude & Altitude controller/3(Z ref)
  [Transition] -> Attitude & Altitude controller/4(InTransition)
  Attitude & Altitude controller/1(Roll torque cmd) -> Organize Inputs/2(commanded phi torque)
  Attitude & Altitude controller/2(Pitch torque Cmd) -> Organize Inputs/3(commanded theta torque)
  Attitude & Altitude controller/4(commanded thrust) -> Organize Inputs/5(commanded thrust)
  FlightMode/1 -> Attitude & Altitude controller/5(FlightMode)
  Attitude & Altitude controller/3(Yaw torque Cmd) -> Organize Inputs/4(commanded psi torque)
  [Transition] -> NOT1/1, transition controller/Enable
  [YawRef] -> Mux/3
  Demux1/2 -> [YRef]
  Merge/1 -> Mux/1
  Merge1/1 -> Mux/2
  transition controller/1(Rollcmd) -> Merge/2
  transition controller/2(Pitchcmd) -> Merge1/2
  Horizontal Position Control/1(Roll Cmd) -> Merge/1
  Horizontal Position Control/2(Pitch Cmd) -> Merge1/1

== system auto/Auto1/Scheduler ==
  MotorCommands : Inport
  FlightState : Inport  Port=2  OutDataTypeStr=Enum: flightState
  FixedWingActuators : Inport  Port=3
  " Armed" : EnablePort
  FixedWingScheduler : Subsystem
  Subsystem : Subsystem
  MotorActuatorCommands : Outport  OutputWhenDisabled=reset  InitialOutput=0
  CtrlSurfaceCommands : Outport  Port=2  OutDataTypeStr=Bus: FixedWingCtrlBus  OutputWhenDisabled=reset  InitialOutput=0  VectorParamsAs1DForOutWhenUnconnected=off
  wires:
  FixedWingScheduler/1(ActuatorControls) -> CtrlSurfaceCommands/1, Subsystem/2(FixedWingActuators)
  FlightState/1 -> Subsystem/1(FlightState), FixedWingScheduler/1(FlightState)
  Subsystem/1(ActuatorControls) -> MotorActuatorCommands/1
  MotorCommands/1 -> Subsystem/3(MotorCommands)
  FixedWingActuators/1 -> FixedWingScheduler/2(FixedWingActuators)

== system auto/Auto/Guidance Mode Selector/GuidanceLogic.WP/Back Transition Guard ==
  note: Set previous waypoint to current location if the UAV has just exited back transition
  Poses : Inport
  FromWP : Inport  Port=2
  Bus Selector : BusSelector  OutputSignals=mode
  Bus Selector1 : BusSelector  OutputSignals=position,params,mode
  Constant : Constant  Value=6
  Equal : RelationalOperator  Operator===  OutDataTypeStr=boolean  RndMeth=Simplest  InputSameDT=off
  Switch : Switch  Criteria=u2 > Threshold  SaturateOnIntegerOverflow=off  InputSameDT=off
  Triggered Subsystem : Subsystem  TreatAsAtomicUnit=on
  Out Bus Element2 : Outport  PortName=PrevWP  Element=mode
  Out Bus Element : Outport  PortName=PrevWP  Element=position
  Out Bus Element1 : Outport  PortName=PrevWP  Element=params
  wires:
  FromWP/1 -> Bus Selector1/1, Bus Selector/1
  Bus Selector/1 -> Equal/2  "<mode>"
  Constant/1 -> Equal/1
  Equal/1 -> Switch/2, Triggered Subsystem/Trigger
  Poses/1 -> Triggered Subsystem/1(Poses)
  Triggered Subsystem/1(HoldPositionValue) -> Switch/1
  Switch/1 -> Out Bus Element/1
  Bus Selector1/2 -> Out Bus Element1/1  "<params>"
  Bus Selector1/3 -> Out Bus Element2/1  "<mode>"
  Bus Selector1/1 -> Switch/3  "<position>"

== system auto/Auto/Guidance Mode Selector/GuidanceLogic.WP/Dist2WP ==
  Pose : Inport
  FromWP : Inport  Port=2
  ToWP : Inport  Port=3
  Bus Selector : BusSelector  OutputSignals=position
  Bus Selector1 : BusSelector  OutputSignals=position
  Demux : Demux  Outputs=[3 1]
  Dot Product : DotProduct  OutDataTypeStr=Inherit: Inherit via internal rule
  Subsystem : Subsystem
  Sum : Sum  Inputs=|-+
  Sum1 : Sum  Inputs=|+-
  Terminator : Terminator
  Dist : Outport
  wires:
  Sum1/1 -> Subsystem/1(V)
  Demux/2 -> Terminator/1
  Bus Selector/1 -> Sum/2, Sum1/1  "<position>"
  Demux/1 -> Sum/1
  Bus Selector1/1 -> Sum1/2  "<position>"
  Sum/1 -> Dot Product/1
  Subsystem/1(V_unit) -> Dot Product/2
  Pose/1 -> Demux/1
  Dot Product/1 -> Dist/1
  ToWP/1 -> Bus Selector/1
  FromWP/1 -> Bus Selector1/1

== system auto/Auto1/Blend Scheduler/BTalpha ==
  States : Inport
  Bus Selector : BusSelector  OutputSignals=airspeed
  Constant : Constant  Value=65
  Gain : Gain  Gain=1/20
  Saturation : Saturate  UpperLimit=1  LowerLimit=0
  Subtract : Sum  Inputs=+-
  alpha : Outport
  wires:
  Constant/1 -> Subtract/1
  Subtract/1 -> Gain/1
  Gain/1 -> Saturation/1
  Saturation/1 -> alpha/1
  States/1 -> Bus Selector/1
  Bus Selector/1 -> Subtract/2  "<airspeed>"

== system auto/Auto1/Blend Scheduler/FTalpha ==
  States : Inport
  1-a : Sum  Inputs=+-
  Bus Selector : BusSelector  OutputSignals=airspeed
  Constant3 : Constant  Value=35
  Constant5 : Constant  Value=Cruise_a
  Gain3 : Gain  Gain=1/10
  Saturation1 : Saturate  UpperLimit=10  LowerLimit=0
  Sum2 : Sum  Inputs=|+-
  alpha : Outport
  wires:
  1-a/1 -> alpha/1
  Bus Selector/1 -> Sum2/1  "<airspeed>"
  Gain3/1 -> 1-a/2
  Sum2/1 -> Saturation1/1
  Saturation1/1 -> Gain3/1
  Constant3/1 -> Sum2/2
  States/1 -> Bus Selector/1
  Constant5/1 -> 1-a/1

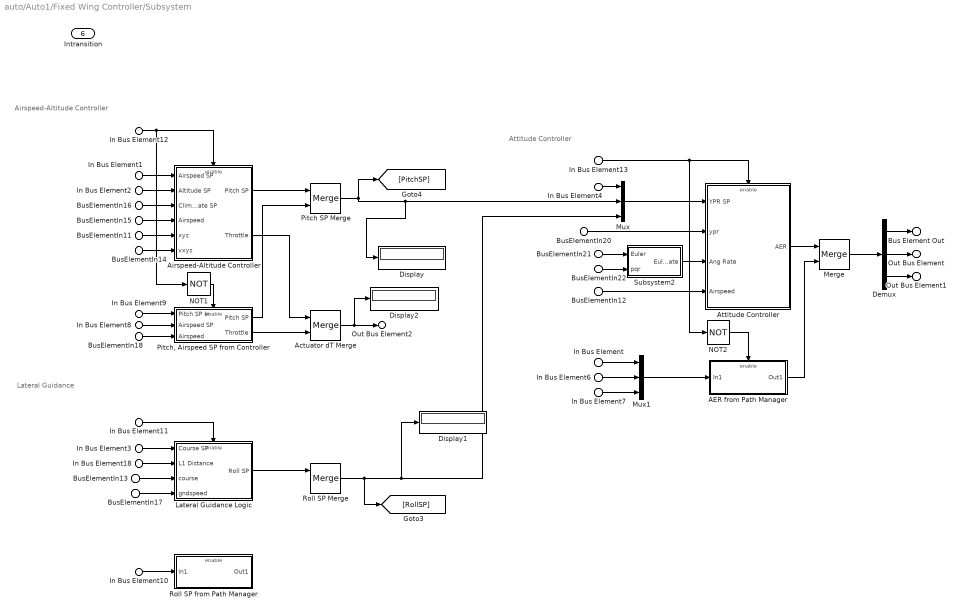
== system auto/Auto1/Fixed Wing Controller/Subsystem ==
  note: Airspeed-Altitude Controller
  note: Lateral Guidance
  note: Attitude Controller
  BusElementIn11 : Inport  PortName=States  Element=Xe
  BusElementIn12 : Inport  PortName=States  Element=airspeed
  BusElementIn15 : Inport  PortName=States  Element=airspeed
  BusElementIn18 : Inport  PortName=States  Element=airspeed
  BusElementIn13 : Inport  PortName=States  Element=course
  BusElementIn16 : Inport  PortName=States  Element=course
  BusElementIn14 : Inport  PortName=States  Element=Ve_ground
  BusElementIn17 : Inport  PortName=States  Element=gndspeed
  BusElementIn20 : Inport  PortName=States  Element=YPR
  BusElementIn21 : Inport  PortName=States  Element=Euler
  BusElementIn22 : Inport  PortName=States  Element=pqr
  In Bus Element11 : Inport  Port=2  PortName=Control Mode  Element=lateralGuidance
  In Bus Element12 : Inport  Port=2  PortName=Control Mode  Element=airspeedAltitude
  In Bus Element13 : Inport  Port=2  PortName=Control Mode  Element=attitude
  In Bus Element1 : Inport  Port=3  PortName=AAC SP  Element=airspeed
  In Bus Element2 : Inport  Port=3  PortName=AAC SP  Element=altitude
  In Bus Element18 : Inport  Port=3  PortName=AAC SP  Element=L1
  In Bus Element3 : Inport  Port=3  PortName=AAC SP  Element=course
  In Bus Element4 : Inport  Port=4  PortName=FixedWingSP  Element=yaw
  In Bus Element9 : Inport  Port=4  PortName=FixedWingSP  Element=pitch
  In Bus Element10 : Inport  Port=4  PortName=FixedWingSP  Element=roll
  In Bus Element8 : Inport  Port=4  PortName=FixedWingSP  Element=airspeed
  In Bus Element : Inport  Port=5  PortName=AERT  Element=aileron
  In Bus Element6 : Inport  Port=5  PortName=AERT  Element=elevator
  In Bus Element7 : Inport  Port=5  PortName=AERT  Element=rudder
  Intransition : Inport  Port=6
  AER from Path Manager : Subsystem  TreatAsAtomicUnit=on
  Actuator dT Merge : Merge
  Airspeed-Altitude Controller : Subsystem
  Attitude Controller : Subsystem
  Demux : Demux  Outputs=3
  Display : Display
  Display1 : Display
  Display2 : Display
  Lateral Guidance Logic : Subsystem
  Merge : Merge
  Mux : Mux  Inputs=3
  Mux1 : Mux  Inputs=3
  NOT1 : Logic  Operator=NOT  IconShape=distinctive  AllPortsSameDT=off  OutDataTypeStr=boolean
  NOT2 : Logic  Operator=NOT  IconShape=distinctive  AllPortsSameDT=off  OutDataTypeStr=boolean
  Pitch SP Merge : Merge
  "Pitch, Airspeed SP from Controller" : Subsystem  TreatAsAtomicUnit=on
  Roll SP Merge : Merge
  Roll SP from Path Manager : Subsystem  TreatAsAtomicUnit=on
  Subsystem2 : Subsystem
  Bus Element Out : Outport  PortName=Actuator  Element=dA
  Out Bus Element : Outport  PortName=Actuator  Element=dE
  Out Bus Element1 : Outport  PortName=Actuator  Element=dR
  Out Bus Element2 : Outport  PortName=Actuator  Element=dT
  wires:
  In Bus Element4/1 -> Mux/1
  Roll SP Merge/1 -> [RollSP], Display1/1, Mux/3
  BusElementIn18/1 -> "Pitch, Airspeed SP from Controller"/3(Airspeed)
  In Bus Element12/1 -> Airspeed-Altitude Controller/Enable, NOT1/1
  In Bus Element3/1 -> Lateral Guidance Logic/1(Course SP)
  Mux1/1 -> AER from Path Manager/1(In1)
  In Bus Element11/1 -> Lateral Guidance Logic/Enable
  Lateral Guidance Logic/1(Roll SP) -> Roll SP Merge/1
  In Bus Element7/1 -> Mux1/3
  Demux/2 -> Out Bus Element/1
  Demux/1 -> Bus Element Out/1
  In Bus Element9/1 -> "Pitch, Airspeed SP from Controller"/1(Pitch SP In)
  Merge/1 -> Demux/1
  In Bus Element18/1 -> Lateral Guidance Logic/2(L1 Distance)
  In Bus Element13/1 -> NOT2/1, Attitude Controller/Enable
  "Pitch, Airspeed SP from Controller"/1(Pitch SP) -> Pitch SP Merge/2
  BusElementIn14/1 -> Airspeed-Altitude Controller/6(vxyz)
  Pitch SP Merge/1 -> Display/1, Mux/2, [PitchSP]
  BusElementIn15/1 -> Airspeed-Altitude Controller/4(Airspeed)
  In Bus Element8/1 -> "Pitch, Airspeed SP from Controller"/2(Airspeed SP)
  BusElementIn13/1 -> Lateral Guidance Logic/3(course)
  Airspeed-Altitude Controller/2(Throttle) -> Actuator dT Merge/1
  BusElementIn16/1 -> Airspeed-Altitude Controller/3(Climb Rate SP)
  In Bus Element1/1 -> Airspeed-Altitude Controller/1(Airspeed SP)
  BusElementIn11/1 -> Airspeed-Altitude Controller/5(xyz)
  BusElementIn12/1 -> Attitude Controller/4(Airspeed)
  In Bus Element2/1 -> Airspeed-Altitude Controller/2(Altitude SP)
  BusElementIn20/1 -> Attitude Controller/2(ypr)
  Mux/1 -> Attitude Controller/1(YPR SP)
  Demux/3 -> Out Bus Element1/1
  BusElementIn21/1 -> Subsystem2/1(Euler)
  Subsystem2/1(Euler Rate) -> Attitude Controller/3(Ang Rate)
  "Pitch, Airspeed SP from Controller"/2(Throttle) -> Actuator dT Merge/2
  Airspeed-Altitude Controller/1(Pitch SP) -> Pitch SP Merge/1
  Attitude Controller/1(AER) -> Merge/1
  AER from Path Manager/1(Out1) -> Merge/2
  In Bus Element/1 -> Mux1/1
  In Bus Element10/1 -> Roll SP from Path Manager/1(In1)
  In Bus Element6/1 -> Mux1/2
  NOT2/1 -> AER from Path Manager/Enable
  BusElementIn22/1 -> Subsystem2/2(pqr)
  Actuator dT Merge/1 -> Display2/1, Out Bus Element2/1
  BusElementIn17/1 -> Lateral Guidance Logic/4(gndspeed)
  NOT1/1 -> "Pitch, Airspeed SP from Controller"/Enable

== system auto/Auto1/Multicopter Controller/Attitude & Altitude controller ==
  Ref Attitude : Inport
  States : Inport  Port=2
  Z ref : Inport  Port=3
  InTransition : Inport  Port=4
  FlightMode : Inport  Port=5
  Altitude Control : Subsystem
  Bus Selector : BusSelector  OutputSignals=RC
  Compare To Constant : simulink/Logic and Bit Operations/Compare To Constant  relop=>  const=1700  OutDataTypeStr=boolean
  Derivative Gain : Subsystem  VariantControl=AttitudeControl==1
  Selector : Selector  InputPortWidth=10  IndexOptions=Index vector (dialog)  Indices=7  OutputSizes=1
  Roll torque cmd : Outport
  Pitch torque Cmd : Outport  Port=2
  Yaw torque Cmd : Outport  Port=3
  commanded thrust : Outport  Port=4
  wires:
  Altitude Control/1(commanded thrust) -> commanded thrust/1
  Derivative Gain/1(Roll torque cmd) -> Roll torque cmd/1
  InTransition/1 -> Altitude Control/3(InTransition)
  Derivative Gain/2(Pitch torque Cmd) -> Pitch torque Cmd/1
  States/1 -> Derivative Gain/2(States), Bus Selector/1, Altitude Control/1(States)
  Derivative Gain/3(Yaw torque Cmd) -> Yaw torque Cmd/1
  Z ref/1 -> Altitude Control/2(Z ref)
  FlightMode/1 -> Altitude Control/4(FlightMode)
  Ref Attitude/1 -> Derivative Gain/1(Ref Attitude)
  Selector/1 -> Compare To Constant/1
  Bus Selector/1 -> Selector/1  "<RC>"
  Compare To Constant/1 -> Altitude Control/Enable

== system auto/Auto1/Multicopter Controller/Horizontal Position Control ==
  note: Forward Motion is controlled using Tilt.
      | Lateral Motion occurs using roll.
  XRef : Inport
  YRef : Inport  Port=2
  States : Inport  Port=3
  Enable : EnablePort  ShowOutputPort=on
  Saturation : Saturate  UpperLimit=0.75  LowerLimit=-0.75
  Saturation1 : Saturate  UpperLimit=1  LowerLimit=-0.75
  Signal Conversion : SignalConversion  OverrideOpt=off
  Signal Conversion1 : SignalConversion  OverrideOpt=off
  XY Controller : Subsystem
  Roll Cmd : Outport
  Pitch Cmd : Outport  Port=2
  wires:
  XRef/1 -> XY Controller/1(X_ref)
  YRef/1 -> XY Controller/2(Y_ref)
  States/1 -> XY Controller/3(States)
  XY Controller/1(Forward cmd) -> Saturation1/1
  XY Controller/2(Sideward Cmd) -> Saturation/1
  Saturation1/1 -> Signal Conversion/1
  Saturation/1 -> Signal Conversion1/1
  Signal Conversion/1 -> Pitch Cmd/1
  Signal Conversion1/1 -> Roll Cmd/1
  Enable/1 -> XY Controller/Enable

== system auto/Auto1/Multicopter Controller/Organize Inputs ==
  forward command : Inport
  commanded phi torque : Inport  Port=2
  commanded theta torque : Inport  Port=3
  commanded psi torque : Inport  Port=4
  commanded thrust : Inport  Port=5
  Out Bus Element : Outport  PortName=MixerCommands  Element=w_phi
  Out Bus Element1 : Outport  PortName=MixerCommands  Element=w_theta
  Out Bus Element2 : Outport  PortName=MixerCommands  Element=w_psi
  Out Bus Element3 : Outport  PortName=MixerCommands  Element=w_z
  Out Bus Element4 : Outport  PortName=MixerCommands  Element=l_x
  wires:
  commanded theta torque/1 -> Out Bus Element1/1  "theta"
  commanded psi torque/1 -> Out Bus Element2/1
  commanded thrust/1 -> Out Bus Element3/1
  forward command/1 -> Out Bus Element4/1
  commanded phi torque/1 -> Out Bus Element/1  "phi"

== system auto/Auto1/Multicopter Controller/transition controller ==
  Enable : EnablePort
  Constant : Constant  Value=0
  Constant1 : Constant  Value=0
  Rollcmd : Outport
  Pitchcmd : Outport  Port=2
  wires:
  Constant/1 -> Rollcmd/1
  Constant1/1 -> Pitchcmd/1

== system auto/Auto1/Scheduler/FixedWingScheduler ==
  note: C opyright 2024 The MathWorks, Inc.
  note: Fixed Wing Control Mixer
  FlightState : Inport
  FixedWingActuators : Inport  Port=2  OutDataTypeStr=Bus: FixedWingCtrlBus
  Merge : Merge  Inputs=4
  Switch Case : SwitchCase  CaseConditions={flightState.Hover, flightState.Transition, flightState.FixedWing,flightState.BackTransition}  ShowDefaultCase=off
  Switch Case Action Subsystem : Subsystem  TreatAsAtomicUnit=on
  Switch Case Action Subsystem1 : Subsystem  TreatAsAtomicUnit=on
  Switch Case Action Subsystem2 : Subsystem  TreatAsAtomicUnit=on
  Switch Case Action Subsystem3 : Subsystem  TreatAsAtomicUnit=on
  ActuatorControls : Outport
  wires:
  FlightState/1 -> Switch Case/1
  FixedWingActuators/1 -> Switch Case Action Subsystem2/1(FixedWingActuators), Switch Case Action Subsystem1/1(FixedWingActuators)
  Switch Case/3 -> Switch Case Action Subsystem2/Action
  Switch Case/2 -> Switch Case Action Subsystem1/Action
  Switch Case Action Subsystem3/1(FixedWingControls) -> Merge/4
  Merge/1 -> ActuatorControls/1
  Switch Case Action Subsystem1/1(FixedWingControls) -> Merge/2
  Switch Case/4 -> Switch Case Action Subsystem3/Action
  Switch Case Action Subsystem/1(FixedWingControls) -> Merge/1
  Switch Case/1 -> Switch Case Action Subsystem/Action
  Switch Case Action Subsystem2/1(FixedWingControls) -> Merge/3

== system auto/Auto1/Scheduler/Subsystem ==
  note: C opyright 2024 The MathWorks, Inc.
  note: Multicopter Control Mixer
  FlightState : Inport
  FixedWingActuators : Inport  Port=2
  MotorCommands : Inport  Port=3
  Actuator To Voltage : Subsystem
  Merge : Merge  Inputs=4
  Switch Case : SwitchCase  CaseConditions={flightState.Hover, flightState.Transition, flightState.FixedWing,flightState.BackTransition}  ShowDefaultCase=off
  Switch Case Action Subsystem : Subsystem  TreatAsAtomicUnit=on
  Switch Case Action Subsystem1 : Subsystem  TreatAsAtomicUnit=on
  Switch Case Action Subsystem2 : Subsystem  TreatAsAtomicUnit=on
  Switch Case Action Subsystem3 : Subsystem  TreatAsAtomicUnit=on
  ActuatorControls : Outport  OutDataTypeStr=Bus: FCCData
  wires:
  Switch Case/4 -> Switch Case Action Subsystem3/Action
  MotorCommands/1 -> Switch Case Action Subsystem3/1(MixerCommands), Switch Case Action Subsystem/1(MixerCommands), Switch Case Action Subsystem1/1(MixerCommands)
  FlightState/1 -> Switch Case/1
  Switch Case Action Subsystem3/1(Actuator) -> Merge/4
  FixedWingActuators/1 -> Switch Case Action Subsystem2/1(FixedWingCtrlBus)
  Switch Case/3 -> Switch Case Action Subsystem2/Action
  Switch Case/2 -> Switch Case Action Subsystem1/Action
  Switch Case Action Subsystem1/1(Actuator) -> Merge/2
  Switch Case/1 -> Switch Case Action Subsystem/Action
  Switch Case Action Subsystem2/1(Actuator) -> Merge/3
  Switch Case Action Subsystem/1(Actuator) -> Merge/1
  Merge/1 -> Actuator To Voltage/1(Motor Commands)
  Actuator To Voltage/1(Actuator) -> ActuatorControls/1

== system auto/Auto/Guidance Mode Selector/GuidanceLogic.WP/Back Transition Guard/Triggered Subsystem ==
  Poses : Inport
  Trigger : TriggerPort  VariantControl=(inherit)
  Reshape : Reshape  OutputDimensionality=Customize  OutputDimensions=[3,1]
  Selector : Selector  InputPortWidth=4  IndexOptions=Index vector (dialog)  Indices=[1 2 3]  OutputSizes=1
  HoldPositionValue : Outport
  wires:
  Poses/1 -> Selector/1
  Selector/1 -> Reshape/1
  Reshape/1 -> HoldPositionValue/1

== system auto/Auto/Guidance Mode Selector/GuidanceLogic.WP/Dist2WP/Subsystem ==
  V : Inport
  Dot Product1 : DotProduct  OutDataTypeStr=Inherit: Inherit via internal rule
  Product : Product  Inputs=*/
  Saturation : Saturate  UpperLimit=inf  LowerLimit=0.00001
  Sqrt : Sqrt
  V_unit : Outport
  wires:
  V/1 -> Dot Product1/2, Dot Product1/1, Product/1
  Sqrt/1 -> Product/2
  Dot Product1/1 -> Saturation/1
  Saturation/1 -> Sqrt/1
  Product/1 -> V_unit/1

== system auto/Auto1/Fixed Wing Controller/Subsystem/AER from Path Manager ==
  In1 : Inport
  Enable : EnablePort
  Out1 : Outport
  wires:
  In1/1 -> Out1/1
